simulink model "completed_microinverter_setup"  (R2022a)
settings: Solver=FixedStepDiscrete  StartTime=0.0  StopTime=2  FixedStep=Ts  RelTol=1e-3
InitFcn:
  | Ts=1e-6;
  | Tcs=1e-4;
values from neighbouring files (symbols this model uses):
  C1_filter = 2e-6    (= 2e-06)    [q4.m]
  C_filter = 100e-6    (= 0.0001)    [q1.m]    (also in q2.m; q4.m = 2e-06)
  f_center = 50    [q4.m]
  F_switch = 1e3    (= 1000)    [q1.m]
  Ki_current = L_filter*Wn^2    (= 15791.3670417)    [q1.m]    (also in q2.m = 63165.468167; q4.m = 493.480220054)
  Ki_pll = (Wn^2) / A    (= 394784.176044)    [q1.m]    (also in q4.m = 1579136.70417)
  Ki_power = 100    [q4.m]
  Ki_voltage = C_filter*Wn^2    (= 3.55305758439)    [q1.m]    (also in q4.m = 0.0710611516878)
  Kp_current = 2*L_filter*DF*Wn    (= 110.584061406)    [q1.m]    (also in q2.m = 71.0753921948; q4.m = 5.49778714378)
  Kp_pll = 2*DF / sqrt(A/Ki_pll)    [q1.m]    (also in q4.m = 2*DF / sqrt(1/Ki_pll))
  Kp_power = 0    [q4.m]
  Kp_voltage = 2*C_filter*DF*Wn    (= 0.0565486677646)    [q1.m]    (also in q4.m = 0.00791681348705)
  L1_filter = 1.5e-3    (= 0.0015)    [q4.m]
  L2_filter = 1.0e-3    (= 0.001)    [q4.m]
  L_filter = 40e-3    (= 0.04)    [q1.m]    (also in q2.m; q4.m = 0.00125)
  L_load = sqrt((R_load * V_rms^2)/P_load - R_load^2) / w    [q1.m]    (also in q4.m)
  R_load = (V_rms^2) * (pf_load^2) / P_load    (= 43.32)    [q1.m]    (also in q4.m)
  Rd_filter = 0.2    [q4.m]
  Tes = 20*Ts    (= 2e-05)    [q1.m]    (also in q4.m)
  V_dc = sqrt(2) * sqrt(3) * V_rms    [q1.m]    (also in q4.m = V_rms * sqrt(3) * sqrt(2))
undefined symbols (not defined in the file or in its folder): DiscIntNeverNeededParam
libraries: ee_lib x111, nesl_utility x28, fl_lib x23, spsabctodq0Lib x11, dspindex x3, spsTriangleGeneratorLib x2, spsdq0toabcLib x2
(part 1 of 4)
settings Model: VariantFading=off  Creator=Kevin  LastModifiedBy=acidi
settings SolverCC: AlgebraicLoopSolver=TrustRegion
settings DebuggingCC: UnconnectedInputMsg=warning  UnconnectedOutputMsg=warning  UnconnectedLineMsg=warning  SFMachineParentedDataDiag=warning

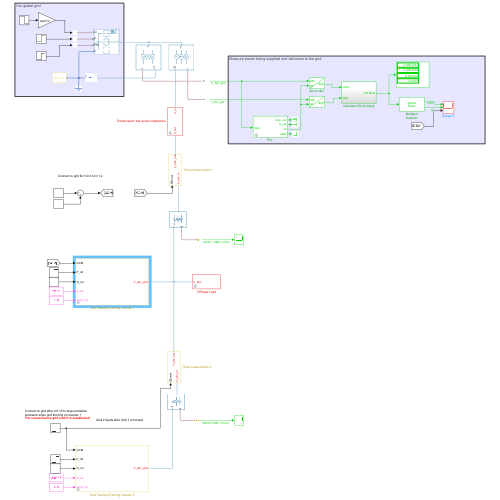
[thumbnail: Simulink's stored preview of the top-level diagram]
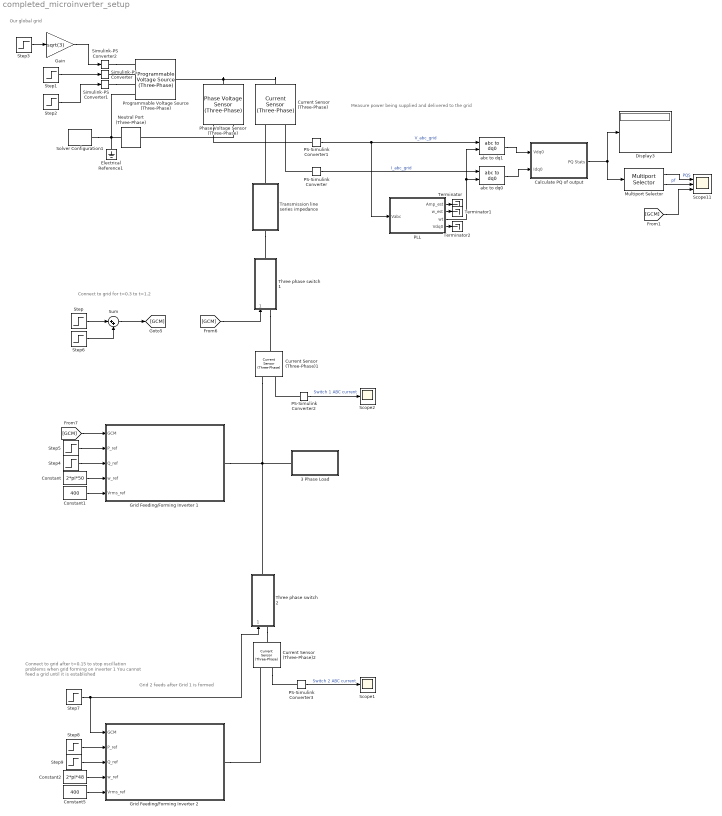
== system completed_microinverter_setup ==
  note: Grid 2 feeds after Grid 1 is formed
  note: Our global grid
  note: Measure power being supplied and delivered to the grid
  note: Connect to grid for t=0.3 to t=1.2
  note: Connect to grid after t=0.15 to stop oscillation problems when grid forming on inverter 1
      | You cannot feed a grid until it is established
  3 Phase Load : Subsystem  mask{R=R_load, L=L_load}
  Calculate PQ of output : Subsystem
  Constant : Constant  Value=2*pi*50
  Constant1 : Constant  Value=400
  Constant2 : Constant  Value=2*pi*48
  Constant5 : Constant  Value=400
  Current Sensor (Three-Phase) : ee_lib/Sensors & Transducers/Current Sensor (Three-Phase)
  Current Sensor (Three-Phase)1 : ee_lib/Sensors & Transducers/Current Sensor (Three-Phase)
  Current Sensor (Three-Phase)2 : ee_lib/Sensors & Transducers/Current Sensor (Three-Phase)
  Display3 : Display
  Electrical Reference1 : fl_lib/Electrical/Electrical Elements/Electrical Reference
      settings: SourceProductBaseCode=PW,SS,VE
  Gain : Gain  Gain=sqrt(3)
  Grid Feeding/Forming Inverter 1 : Subsystem  mask{Ts=Ts, Tes=Tes, Tcs=Tcs, Ki_pll=Ki_pll, Kp_pll=Kp_pll, f_center=f_center, L1_filter=L1_filter, L2_filter=L2_filter, C1_filter=C1_filter, Rd_filter=Rd_filter, C_filter=C_filter, L_filter=L_filter, Ki_current=Ki_current, Kp_current=Kp_current, Ki_voltage=Ki_voltage, Kp_voltage=Kp_voltage, Ki_power=Ki_power, Kp_power=Kp_power}
      mask DialogControl Container5 Prompt: Simulation constants
      mask DialogControl Container6 Prompt: Three Phase PLL
      mask DialogControl ParameterGroupVar Prompt: LCL inverter filter
      mask DialogControl Container3 Prompt: Controller Parameters
      mask DialogControl Container4 Prompt: Current controller
      mask DialogControl Container7 Prompt: Voltage Controller
      mask DialogControl Container8 Prompt: Power Controller
  Grid Feeding/Forming Inverter 2 : Subsystem  mask{Ts=Ts, Tes=Tes, Tcs=Tcs, Ki_pll=Ki_pll, Kp_pll=Kp_pll, f_center=f_center, L1_filter=L1_filter, L2_filter=L2_filter, C1_filter=C1_filter, Rd_filter=Rd_filter, C_filter=C_filter, L_filter=L_filter, Ki_current=Ki_current, Kp_current=Kp_current, Ki_voltage=Ki_voltage, Kp_voltage=Kp_voltage, Ki_power=Ki_power, Kp_power=Kp_power}
      mask DialogControl Container5 Prompt: Simulation constants
      mask DialogControl Container6 Prompt: Three Phase PLL
      mask DialogControl ParameterGroupVar Prompt: LCL inverter filter
      mask DialogControl Container3 Prompt: Controller Parameters
      mask DialogControl Container4 Prompt: Current controller
      mask DialogControl Container7 Prompt: Voltage Controller
      mask DialogControl Container8 Prompt: Power Controller
  Multiport Selector : dspindex/Multiport Selector  rowsOrCols=Rows  idxCellArray={ [1 2 3], 4 }  idxErrMode=Clip Index
  Neutral Port (Three-Phase) : ee_lib/Connectors & References/Neutral Port (Three-Phase)  G_parasitic=1e-12 1/Ohm
      settings: SourceProductBaseCode=PS  InternalSimscapePortConfiguration="{\"Bottom\":[],\"Left\":[{\"id\":\"N\",\"label\":\"~\",\"type\":\"foundation.electrical.three_phase\"}],\"Right\":[{\"id\":\"n\",\"label\":\"n\",\"type\":\"foundation.electrical.electrical\"}],\"Top\":[]}"
  PLL : Subsystem  mask{Ts=Tcs, Ki=Ki_pll, Kp=Kp_pll, f_center=f_center}
      mask DialogControl Container1 Prompt: Parameters
  PS-Simulink Converter{,1..3} (4 alike) : nesl_utility/PS-Simulink Converter  PhysicalDomain=network_engine_domain  SubClassName=ps_output  LeftPortType=input  RightPortType=output  PseudoPeriodic=off  Frequencies=[]  VectorFormat=inherit  Unit=inherit  AffineConversion=off
      settings: SourceProductBaseCode=SS,PW,VE
  Phase Voltage Sensor (Three-Phase) : ee_lib/Sensors & Transducers/Phase Voltage Sensor (Three-Phase)
      settings: SourceProductBaseCode=PS
  Programmable Voltage Source (Three-Phase) : ee_lib/Sources/Programmable Voltage Source (Three-Phase)  magnitude_type=ee.enum.timechanging.external  vline_rms=230*sqrt(3) V  magn_ramp=1 V/s  magn_step=-230*sqrt(3)*0.8 V  magn_modu_magn=1 V  magn_modu_freq=1 Hz  magn_t1=1.2 s  magn_t2=1.6 s  frequency_type=ee.enum.timechanging.external  freq=50 Hz  freq_ramp=1 Hz/s  freq_step=1 Hz  freq_modu_magn=1 Hz  freq_modu_freq=1 Hz  freq_t1=1 s  freq_t2=2 s  phase_type=ee.enum.timechanging.external  shift=45 deg  phase_ramp=1 deg/s  phase_step=15 deg  phase_modu_magn=1 deg  phase_modu_freq=1 Hz  phase_t1=0.5 s  phase_t2=0.9 s  impedance_option=1  SShortCircuit=1e6 V*A  XR=15  R=0.01 Ohm  L=3.97e-4 H  G_parasitic=0 1/Ohm  harmonic_option=0  harmonic_orders=[5, 7, 11, 13]  harmonic_ratios=[.1, .1, .1, .1]  harmonic_shifts=[0, 0, 0, 0] deg  harmonic_sequences=[1, 1, 1, 1]  harmonic_t1=-inf s  harmonic_t2=inf s  I_specify=off  I_priority=None  I=[ 0 0 0 ] A  I_nominal_specify=off  I_nominal_unit=A  I_nominal_value=1  V_specify=off  V_priority=None  V=[0, 400*sqrt(2/3)*sin(-2/3*pi), 400*sqrt(2/3)*sin(-4/3*pi)] V  V_nominal_specify=off  V_nominal_unit=V  V_nominal_value=1
      settings: SourceProductBaseCode=PS  InternalSimscapePortConfiguration="{\"Bottom\":[],\"Left\":[{\"id\":\"ext_magn\",\"label\":\"M\",\"type\":\"input\"},{\"id\":\"ext_freq\",\"label\":\"F\",\"type\":\"input\"},{\"id\":\"ext_phase\",\"label\":\"Phi\",\"type\":\"input\"},{\"id\":\"n\",\"label\":\"n\",\"type\":\"foundation.electrical.electrical\"}],\"Right\":[{\"id\":\"N\",\"label\":\"~\",\"type\":\"foundation.electrical.three_phase\"}],\"Top\":[]}"
  Scope1 : Scope
  Scope11 : Scope  NumInputPorts=3
  Scope2 : Scope
  Simulink-PS Converter : nesl_utility/Simulink-PS Converter  PhysicalDomain=network_engine_domain  SubClassName=ps_input  LeftPortType=input  RightPortType=output  PseudoPeriodic=off  Frequencies=[]  NoiseDistribution=none  NoiseParameters=[]  Unit=1  AffineConversion=off  FilteringAndDerivatives=provide  SimscapeFilterOrder=1  InputFilterTimeConstant=0.001  UdotUserProvided=0
      settings: SourceProductBaseCode=SS,PW,VE
  Simulink-PS Converter1 : nesl_utility/Simulink-PS Converter  PhysicalDomain=network_engine_domain  SubClassName=ps_input  LeftPortType=input  RightPortType=output  PseudoPeriodic=off  Frequencies=[]  NoiseDistribution=none  NoiseParameters=[]  Unit=1  AffineConversion=off  FilteringAndDerivatives=provide  SimscapeFilterOrder=1  InputFilterTimeConstant=0.001  UdotUserProvided=0
      settings: SourceProductBaseCode=SS,PW,VE
  Simulink-PS Converter2 : nesl_utility/Simulink-PS Converter  PhysicalDomain=network_engine_domain  SubClassName=ps_input  LeftPortType=input  RightPortType=output  PseudoPeriodic=off  Frequencies=[]  NoiseDistribution=none  NoiseParameters=[]  Unit=1  AffineConversion=off  FilteringAndDerivatives=provide  SimscapeFilterOrder=1  InputFilterTimeConstant=0.001  UdotUserProvided=0
      settings: SourceProductBaseCode=SS,PW,VE
  Solver Configuration1 : nesl_utility/Solver Configuration  PhysicalDomain=network_engine_domain  SubClassName=solver  LeftPortType=input  RightPortType=generic  Tones=[]  Harmonics=[]  SimulateNoise=off  Profile=off  UseLocalSampling=off  EnableSwitchedLinearOptims=on  FrequencyDomain=off  UseCCode=off  RelTol=0.001  AbsTol=1e-06  MinStep=1e-09  ToWorkspace=off  RevertToSquareIcSolve=off  NumHomotopyIterations=100  PhasorMode=off  PhasorModeNumHarmonics=1  IndexReductionMethod=DerivativeReplacement  DoDC=off  ResidualTolerance=1e-09  UseLocalSolver=on  LocalSolverChoice=NE_BACKWARD_EULER_ADVANCER  LocalSolverSampleTime=Tcs  DoFixedCost=off  MaxNonlinIter=3  MaxModeIter=2  ComputeImpulses=off  ImpulseIterations=2  LinearAlgebra=auto  LinearAlgebraNumThread=0  EquationFormulation=NE_TIME_EF  DelaysMemoryBudget=1024  AutomaticFiltering=off  FilteringTimeConstant=0.001  PartitionStorageMethod=AS_NEEDED  PartitionMemoryBudget=1024  PartitionMethod=ROBUST
      settings: SourceProductBaseCode=SS,PW,VE
  Step : Step  Time=0.3  SampleTime=0
  Step1 : Step  Time=0.4  Before=50  After=53  SampleTime=0
  Step2 : Step  Time=0.6  After=15 * pi/180  SampleTime=0
  Step3 : Step  Time=0.8  Before=400  After=400*0.6  SampleTime=0
  Step4 : Step  Time=0.5  Before=6000  After=-2000  SampleTime=0
  Step5 : Step  Time=0.7  Before=7000  After=15000  SampleTime=0
  Step6 : Step  Time=1.2  After=-1  SampleTime=0
  Step7 : Step  Time=0.15  SampleTime=0
  Step8 : Step  Time=1.4  Before=1000  After=15000  SampleTime=0
  Step9 : Step  Time=1.6  Before=-3000  After=4500  SampleTime=0
  Sum : Sum  Inputs=|++
  Terminator : Terminator
  Terminator1 : Terminator
  Terminator2 : Terminator
  Three phase switch 1 : Subsystem  mask{R_opened=1e9, R_closed=1e-3}
  Three phase switch 2 : Subsystem  mask{R_opened=1e9, R_closed=1e-3}
  Transmission line series impedance : Subsystem  mask{R=100e-3, L=1e-3}
  abc to dq0 : spsabctodq0Lib/abc to dq0  Alignment=90 degrees behind phase A axis
  abc to dq1 : spsabctodq0Lib/abc to dq0  Alignment=90 degrees behind phase A axis
  wires:
  Step1/1 -> Simulink-PS Converter/1
  Step2/1 -> Simulink-PS Converter1/1
  Step3/1 -> Gain/1
  Gain/1 -> Simulink-PS Converter2/1
  [GCM] -> Grid Feeding/Forming Inverter 1/1(GCM)
  Step5/1 -> Grid Feeding/Forming Inverter 1/2(P_ref)
  Step4/1 -> Grid Feeding/Forming Inverter 1/3(Q_ref)
  Constant/1 -> Grid Feeding/Forming Inverter 1/4(w_ref)
  Constant1/1 -> Grid Feeding/Forming Inverter 1/5(Vrms_ref)
  PS-Simulink Converter2/1 -> Scope2/1  "Switch 1 ABC current"
  [GCM] -> Three phase switch 1/1(Control)
  Step7/1 -> Grid Feeding/Forming Inverter 2/1(GCM), Three phase switch 2/1(Control)
  Step8/1 -> Grid Feeding/Forming Inverter 2/2(P_ref)
  Step9/1 -> Grid Feeding/Forming Inverter 2/3(Q_ref)
  Step/1 -> Sum/1
  Step6/1 -> Sum/2
  Constant2/1 -> Grid Feeding/Forming Inverter 2/4(w_ref)
  Constant5/1 -> Grid Feeding/Forming Inverter 2/5(Vrms_ref)
  Calculate PQ of output/1(PQ Stats) -> Multiport Selector/1, Display3/1
  Multiport Selector/1 -> Scope11/1  "PQS"
  Multiport Selector/2 -> Scope11/2  "pf"
  PS-Simulink Converter/1 -> abc to dq0/1  "I_abc_grid"
  PS-Simulink Converter1/1 -> PLL/1(Vabc), abc to dq1/1  "V_abc_grid"
  PLL/3(wt) -> abc to dq1/2, abc to dq0/2
  abc to dq1/1 -> Calculate PQ of output/1(Vdq0)
  abc to dq0/1 -> Calculate PQ of output/2(Idq0)
  [GCM] -> Scope11/3
  PLL/1(Amp_est) -> Terminator/1
  PLL/2(w_est) -> Terminator1/1
  PLL/4(Vdq0) -> Terminator2/1
  PS-Simulink Converter3/1 -> Scope1/1  "Switch 2 ABC current"
  Sum/1 -> [GCM]
  connections:
  Simulink-PS Converter/RConn1 -- Programmable Voltage Source (Three-Phase)/LConn2
  Simulink-PS Converter2/RConn1 -- Programmable Voltage Source (Three-Phase)/LConn1
  Programmable Voltage Source (Three-Phase)/LConn4 -- Electrical Reference1/LConn1 -- Neutral Port (Three-Phase)/RConn1 -- Solver Configuration1/RConn1
  Simulink-PS Converter1/RConn1 -- Programmable Voltage Source (Three-Phase)/LConn3
  Phase Voltage Sensor (Three-Phase)/LConn1 -- Current Sensor (Three-Phase)/LConn1 -- Programmable Voltage Source (Three-Phase)/RConn1
  Grid Feeding/Forming Inverter 1/RConn1 -- Three phase switch 2/RConn1 -- Current Sensor (Three-Phase)1/RConn2 -- 3 Phase Load/LConn1
  Transmission line series impedance/RConn1 -- Three phase switch 1/RConn1
  Grid Feeding/Forming Inverter 2/RConn1 -- Current Sensor (Three-Phase)2/RConn2
  Phase Voltage Sensor (Three-Phase)/RConn2 -- Neutral Port (Three-Phase)/LConn1
  Transmission line series impedance/LConn1 -- Current Sensor (Three-Phase)/RConn2
  PS-Simulink Converter/LConn1 -- Current Sensor (Three-Phase)/RConn1
  PS-Simulink Converter1/LConn1 -- Phase Voltage Sensor (Three-Phase)/RConn1
  Three phase switch 1/LConn1 -- Current Sensor (Three-Phase)1/LConn1
  PS-Simulink Converter2/LConn1 -- Current Sensor (Three-Phase)1/RConn1
  Three phase switch 2/LConn1 -- Current Sensor (Three-Phase)2/LConn1
  Current Sensor (Three-Phase)2/RConn1 -- PS-Simulink Converter3/LConn1

== system completed_microinverter_setup/3 Phase Load ==
  Inductor3 : ee_lib/Passive/Inductor  l=L H  enable_L_tol=0  L_tol=20  tol_distribution=1  nSigma=4  r=0 Ohm  g=1e-9 1/Ohm  enable_operating_limits=0  operating_limit_action=2  max_working_current=1 A  power_rating=1 W  enable_faults=0  fault_action=1  lambdaPercent=50  k_faulted=0.9999  turnsShort=0  openCct=0  groundShort=0  groundShortG=0 1/Ohm  tau_fault=1e-3 s  enable_temporal_fault=0  t_fault=1 s  enable_behavioral_fault=0  max_permissible_voltage=100 V  n_fail_on_voltage=1  max_permissible_current=1 A  t_fail_on_current=1 s  i_L_specify=off  i_L_priority=High  i_L=0 A  i_L_nominal_specify=off  i_L_nominal_unit=A  i_L_nominal_value=1
  Inductor4 : ee_lib/Passive/Inductor  l=L H  enable_L_tol=0  L_tol=20  tol_distribution=1  nSigma=4  r=0 Ohm  g=1e-9 1/Ohm  enable_operating_limits=0  operating_limit_action=2  max_working_current=1 A  power_rating=1 W  enable_faults=0  fault_action=1  lambdaPercent=50  k_faulted=0.9999  turnsShort=0  openCct=0  groundShort=0  groundShortG=0 1/Ohm  tau_fault=1e-3 s  enable_temporal_fault=0  t_fault=1 s  enable_behavioral_fault=0  max_permissible_voltage=100 V  n_fail_on_voltage=1  max_permissible_current=1 A  t_fail_on_current=1 s  i_L_specify=off  i_L_priority=High  i_L=0 A  i_L_nominal_specify=off  i_L_nominal_unit=A  i_L_nominal_value=1
  Inductor5 : ee_lib/Passive/Inductor  l=L H  enable_L_tol=0  L_tol=20  tol_distribution=1  nSigma=4  r=0 Ohm  g=1e-9 1/Ohm  enable_operating_limits=0  operating_limit_action=2  max_working_current=1 A  power_rating=1 W  enable_faults=0  fault_action=1  lambdaPercent=50  k_faulted=0.9999  turnsShort=0  openCct=0  groundShort=0  groundShortG=0 1/Ohm  tau_fault=1e-3 s  enable_temporal_fault=0  t_fault=1 s  enable_behavioral_fault=0  max_permissible_voltage=100 V  n_fail_on_voltage=1  max_permissible_current=1 A  t_fail_on_current=1 s  i_L_specify=off  i_L_priority=High  i_L=0 A  i_L_nominal_specify=off  i_L_nominal_unit=A  i_L_nominal_value=1
  Phase Splitter1 : ee_lib/Connectors & References/Phase Splitter
      settings: SourceProductBaseCode=PS
  Resistor : ee_lib/Passive/Resistor  R=R Ohm  enable_R_tol=0  R_tol=5  tol_distribution=1  nSigma=4  enable_operating_limits=0  operating_limit_action=2  max_working_voltage=100 V  power_rating=1 W  enable_faults=0  fault_action=1  R_faulted=inf Ohm  enable_temporal_fault=0  t_fault=1 s  enable_behavioral_fault=0  max_permissible_current=1 A  t_fail_on_current=1 s  noise_mode=0  sample_time=1e-3 s  repeatability=1  auto_seed=2348838240  user_seed=0  Tdevice=25 degC  power_derating_T1=70 degC  power_derating_T2=155 degC  operating_temperature_range_vec=[-50, 150] degC  alpha=3.93e-3 1/K  Tmeas=25 degC  thermal_mass=100 J/K  temperature_specify=off  temperature_priority=High  temperature=298.15 K  temperature_nominal_specify=off  temperature_nominal_unit=K  temperature_nominal_value=1
  Resistor1 : ee_lib/Passive/Resistor  R=R Ohm  enable_R_tol=0  R_tol=5  tol_distribution=1  nSigma=4  enable_operating_limits=0  operating_limit_action=2  max_working_voltage=100 V  power_rating=1 W  enable_faults=0  fault_action=1  R_faulted=inf Ohm  enable_temporal_fault=0  t_fault=1 s  enable_behavioral_fault=0  max_permissible_current=1 A  t_fail_on_current=1 s  noise_mode=0  sample_time=1e-3 s  repeatability=1  auto_seed=4112460543  user_seed=0  Tdevice=25 degC  power_derating_T1=70 degC  power_derating_T2=155 degC  operating_temperature_range_vec=[-50, 150] degC  alpha=3.93e-3 1/K  Tmeas=25 degC  thermal_mass=100 J/K  temperature_specify=off  temperature_priority=High  temperature=298.15 K  temperature_nominal_specify=off  temperature_nominal_unit=K  temperature_nominal_value=1
  Resistor2 : ee_lib/Passive/Resistor  R=R Ohm  enable_R_tol=0  R_tol=5  tol_distribution=1  nSigma=4  enable_operating_limits=0  operating_limit_action=2  max_working_voltage=100 V  power_rating=1 W  enable_faults=0  fault_action=1  R_faulted=inf Ohm  enable_temporal_fault=0  t_fault=1 s  enable_behavioral_fault=0  max_permissible_current=1 A  t_fail_on_current=1 s  noise_mode=0  sample_time=1e-3 s  repeatability=1  auto_seed=4144164703  user_seed=0  Tdevice=25 degC  power_derating_T1=70 degC  power_derating_T2=155 degC  operating_temperature_range_vec=[-50, 150] degC  alpha=3.93e-3 1/K  Tmeas=25 degC  thermal_mass=100 J/K  temperature_specify=off  temperature_priority=High  temperature=298.15 K  temperature_nominal_specify=off  temperature_nominal_unit=K  temperature_nominal_value=1
  V_abc : PMIOPort  Side=Left
  connections:
  Resistor2/LConn1 -- Inductor5/RConn1
  Phase Splitter1/RConn1 -- Inductor3/LConn1
  Phase Splitter1/RConn3 -- Inductor5/LConn1
  Resistor/RConn1 -- Resistor2/RConn1 -- Resistor1/RConn1
  Resistor1/LConn1 -- Inductor4/RConn1
  Phase Splitter1/RConn2 -- Inductor4/LConn1
  Resistor/LConn1 -- Inductor3/RConn1
  V_abc/RConn1 -- Phase Splitter1/LConn1

== system completed_microinverter_setup/Calculate PQ of output ==
  note: Reorient Vdq0 so that Uq = 0, Ud = defined
  Vdq0 : Inport
  Idq0 : Inport  Port=2
  Atan2 : Trigonometry  Operator=atan2
  Cos : Trigonometry  Operator=cos
  Demux : Demux  Outputs=3
  Demux1 : Demux  Outputs=2
  Gain2 : Gain  Gain=3/2
  MatrixMultiply1 : Product  Multiplication=Matrix(*)
  MatrixMultiply2 : Product  Multiplication=Matrix(*)
  Mux : Mux
  Product : Product
  Product2 : Product
  Selector : Selector  InputPortWidth=3  IndexOptions=Index vector (dialog)  Indices=[1 2]  OutputSizes=1
  Selector1 : Selector  InputPortWidth=3  IndexOptions=Index vector (dialog)  Indices=[1]  OutputSizes=1
  Sign : Signum
  Sqrt : Sqrt
  Square : Math  Operator=square
  Subsystem : Subsystem
  Sum of Elements : Sum  Inputs=+
  Terminator : Terminator
  PQ Stats : Outport
  wires:
  Product2/1 -> Gain2/1
  Square/1 -> Sum of Elements/1
  Gain2/1 -> Demux/1, Selector/1
  Sum of Elements/1 -> Sqrt/1
  Selector/1 -> Square/1, Demux1/1
  Vdq0/1 -> MatrixMultiply1/2, Subsystem/1(Vdq0)
  Subsystem/1(Rotation Matrix) -> MatrixMultiply2/1, MatrixMultiply1/1
  Idq0/1 -> MatrixMultiply2/2
  MatrixMultiply1/1 -> Selector1/1
  MatrixMultiply2/1 -> Product2/2
  Demux/3 -> Terminator/1
  Demux/2 -> Atan2/1  "Q"
  Demux/1 -> Atan2/2  "P"
  Atan2/1 -> Cos/1
  Demux1/1 -> Mux/1  "P"
  Demux1/2 -> Sign/1, Mux/2  "Q"
  Sqrt/1 -> Mux/3  "|S|"
  Product/1 -> Mux/4  "pf"
  Mux/1 -> PQ Stats/1
  Selector1/1 -> Product2/1
  Sign/1 -> Product/1
  Cos/1 -> Product/2  "pf"

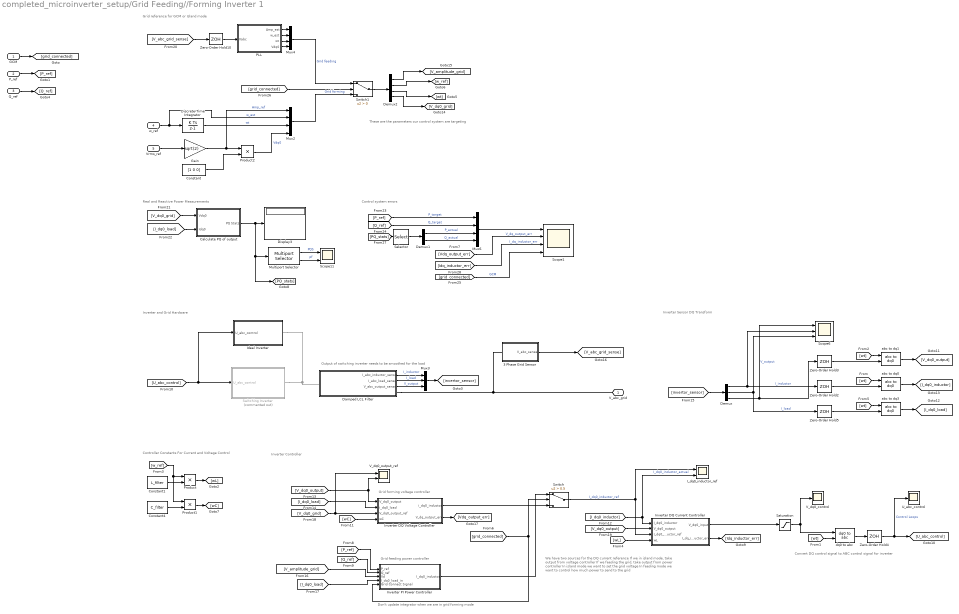
== system completed_microinverter_setup/Grid Feeding//Forming Inverter 1 ==
  note: Grid forming voltage controller
  note: Output of switching inverter needs to be smoothed for the load
  note: These are the parameters our control system are targeting
  note: Don't update integrator when we are in grid forming mode
  note: We have two sources for the DQ current reference
      | If we in island mode, take output from voltage controller
      | If we feeding the grid, take output from power controller
      |
      | In island mode we want to set the grid voltage
      | In feeding mode we want to control how much power to send to the grid
  note: Convert DQ control signal to ABC control signal for inverter
  note: Control system errors
  note: Grid reference for GCM or Island mode
  note: Real and Reactive Power Measurements
  note: Inverter and Grid Hardware
  note: Inverter Sensor DQ Transform
  note: Inverter Controller
  note: Controller Constants For Current and Voltage Control
  note: Grid feeding power controller
  GCM : Inport
  P_ref : Inport  Port=2
  Q_ref : Inport  Port=3
  w_ref : Inport  Port=4
  Vrms_ref : Inport  Port=5
  3 Phase Grid Sensor : Subsystem  mask{R=10e3}
  Calculate PQ of output : Subsystem
  Constant : Constant  Value=[1 0 0]
  Constant1 : Constant  Value=L_filter
  Constant4 : Constant  Value=C_filter
  Damped LCL Filter : Subsystem  mask{L1=L1_filter, L2=L2_filter, C=C1_filter, Rd=Rd_filter, Ts=Tcs}
  Demux : Demux  Outputs=3
  Demux1 : Demux  Outputs=2
  Demux2 : Demux
  Discrete-Time Integrator : DiscreteIntegrator  SampleTime=Tcs  UpperSaturationLimit=2*pi*10  LowerSaturationLimit=-2*pi*10  ICPrevOutput=DiscIntNeverNeededParam  ICPrevScaledInput=DiscIntNeverNeededParam
  Display3 : Display
  Gain : Gain  Gain=sqrt(2)
  I_dq0_inductor_ref : Scope  NumInputPorts=2
  Ideal Inverter : Subsystem
  Inverter DQ Current Controller : Subsystem  mask{Kp=Kp_current, Ki=Ki_current, Ts=Tcs}
  Inverter DQ Voltage Controller : Subsystem  mask{Kp=Kp_voltage, Ki=Ki_voltage, Ts=Tcs}
  Inverter PI Power Controller : Subsystem  mask{Ki=Ki_power, Kp=Kp_power, Ts=Tcs}
  Multiport Selector : dspindex/Multiport Selector  rowsOrCols=Rows  idxCellArray={ [1 2 3], 4 }  idxErrMode=Clip Index
  Mux2 : Mux
  Mux3 : Mux  Inputs=3
  Mux4 : Mux
  Mux6 : Mux
  PLL : Subsystem  mask{Ts=Tcs, Ki=Ki_pll, Kp=Kp_pll, f_center=f_center}
      mask DialogControl Container1 Prompt: Parameters
  Product : Product
  Product1 : Product
  Product2 : Product
  Saturation : Saturate  UpperLimit=600  LowerLimit=-600
  Scope1 : Scope  NumInputPorts=4
  Scope11 : Scope  NumInputPorts=2
  Scope6 : Scope  NumInputPorts=3
  Selector : Selector  InputPortWidth=4  IndexOptions=Index vector (dialog)  Indices=[1 2]  OutputSizes=1
  Switch : Switch  Criteria=u2 > Threshold  Threshold=0.5  SaturateOnIntegerOverflow=off  InputSameDT=off
  Switch1 : Switch  Criteria=u2 > Threshold  SaturateOnIntegerOverflow=off  InputSameDT=off
  Switching Inverter : Subsystem  Commented=on  TreatAsAtomicUnit=on  mask{V_dc=V_dc, F_switch=F_switch, Ts=Tes}
  U_abc_control : Scope
  V_dq0_control : Scope
  V_dq0_output_ref : Scope  NumInputPorts=2
  Zero-Order Hold{2..5,10} (5 alike) : ZeroOrderHold  SampleTime=Tcs
  abc to dq0 : spsabctodq0Lib/abc to dq0  Alignment=Aligned with phase A axis
  abc to dq1 : spsabctodq0Lib/abc to dq0  Alignment=Aligned with phase A axis
  abc to dq3 : spsabctodq0Lib/abc to dq0  Alignment=Aligned with phase A axis
  dq0 to abc : spsdq0toabcLib/dq0 to abc  Alignment=Aligned with phase A axis
  V_abc_grid : PMIOPort  Side=Right
  wires:
  abc to dq1/1 -> [V_dq0_output]
  [w_ref] -> Product/1, Product1/1
  Constant1/1 -> Product/2
  Product1/1 -> [wC]
  [wt] -> abc to dq1/2
  Zero-Order Hold4/1 -> [U_abc_control], U_abc_control/1  "Control Loops"
  [wC] -> Inverter DQ Voltage Controller/4(wC)
  Switch/1 -> I_dq0_inductor_ref/1, Inverter DQ Current Controller/3(I_dq0_inductor_ref)  "I_dq0_inductor_ref"
  Inverter DQ Current Controller/1(V_dq0_input) -> Saturation/1
  [wt] -> dq0 to abc/2
  Constant4/1 -> Product1/2
  [wL] -> Inverter DQ Current Controller/4(wL)
  Product/1 -> [wL]
  dq0 to abc/1 -> Zero-Order Hold4/1
  [wt] -> abc to dq0/2
  [wt] -> abc to dq3/2
  Demux/2 -> Scope6/3, Zero-Order Hold5/1  "I_load"
  Demux/1 -> Scope6/2, Zero-Order Hold2/1  "I_inductor"
  Demux/3 -> Scope6/1, Zero-Order Hold3/1  "V_output"
  Zero-Order Hold10/1 -> PLL/1(Vabc)
  Saturation/1 -> dq0 to abc/1, V_dq0_control/1
  Zero-Order Hold2/1 -> abc to dq0/1
  Damped LCL Filter/1(I_abc_inductor_sense) -> Mux3/1  "I_inductor"
  Damped LCL Filter/2(I_abc_load_sense) -> Mux3/2  "I_load"
  Damped LCL Filter/3(V_abc_output_sense) -> Mux3/3  "V_output"
  Mux3/1 -> [invertor_sensor]
  Zero-Order Hold5/1 -> abc to dq3/1
  [grid_connected] -> Switch/2, Inverter PI Power Controller/5(Grid Connect Signal)
  [P_ref] -> Inverter PI Power Controller/1(P_ref)
  [Q_ref] -> Inverter PI Power Controller/2(Q_ref)
  Calculate PQ of output/1(PQ Stats) -> [PQ_stats], Multiport Selector/1, Display3/1
  Zero-Order Hold3/1 -> abc to dq1/1
  [U_abc_control] -> Ideal Inverter/1(U_abc_control), Switching Inverter/1(U_abc_control)
  [V_dq0_output] -> Inverter DQ Voltage Controller/1(V_dq0_output), V_dq0_output_ref/2
  abc to dq3/1 -> [I_dq0_load]
  abc to dq0/1 -> [I_dq0_inductor]
  [V_amplitude_grid] -> Inverter PI Power Controller/3(Vd)
  [I_dq0_load] -> Inverter PI Power Controller/4(I_dq0_load_in)
  [V_dq0_grid] -> V_dq0_output_ref/1, Inverter DQ Voltage Controller/3(V_dq0_output_ref)
  [I_dq0_load] -> Inverter DQ Voltage Controller/2(i_dq0_load)
  [I_dq0_inductor] -> I_dq0_inductor_ref/2, Inverter DQ Current Controller/1(I_dq0_inductor)  "I_dq0_inductor_actual"
  [V_dq0_output] -> Inverter DQ Current Controller/2(V_dq0_output)
  3 Phase Grid Sensor/1(V_abc_sense) -> [V_abc_grid_sense]
  [V_abc_grid_sense] -> Zero-Order Hold10/1
  [V_dq0_grid] -> Calculate PQ of output/1(Vdq0)
  [I_dq0_load] -> Calculate PQ of output/2(Idq0)
  [invertor_sensor] -> Demux/1
  GCM/1 -> [grid_connected]
  Q_ref/1 -> [Q_ref]
  P_ref/1 -> [P_ref]
  Multiport Selector/1 -> Scope11/1  "PQS"
  Multiport Selector/2 -> Scope11/2  "pf"
  w_ref/1 -> Discrete-Time Integrator/1, Mux2/2  "w_est"
  Discrete-Time Integrator/1 -> Mux2/3  "wt"
  Demux2/1 -> [V_amplitude_grid]
  Demux2/4 -> [V_dq0_grid]
  Demux2/3 -> [wt]
  Demux2/2 -> [w_ref]
  Vrms_ref/1 -> Gain/1
  Gain/1 -> Product2/1, Mux2/1  "Amp_ref"
  Constant/1 -> Product2/2
  Product2/1 -> Mux2/4  "Vdq0"
  PLL/1(Amp_est) -> Mux4/1
  PLL/2(w_est) -> Mux4/2
  PLL/3(wt) -> Mux4/3
  PLL/4(Vdq0) -> Mux4/4
  Switch1/1 -> Demux2/1
  Mux4/1 -> Switch1/1  "Grid feeding"
  [grid_connected] -> Switch1/2
  Mux2/1 -> Switch1/3  "Grid forming"
  [grid_connected] -> Scope1/4  "GCM"
  [PQ_stats] -> Selector/1
  Selector/1 -> Demux1/1
  [P_ref] -> Mux6/1  "P_target"
  [Q_ref] -> Mux6/2  "Q_target"
  Demux1/1 -> Mux6/3  "P_actual"
  Demux1/2 -> Mux6/4  "Q_actual"
  Mux6/1 -> Scope1/1
  [Vdq_output_err] -> Scope1/2  "V_dq_output_err"
  [Idq_inductor_err] -> Scope1/3  "I_dq_inductor_err"
  Inverter DQ Current Controller/2(I_dq_inductor_err) -> [Idq_inductor_err]
  Inverter DQ Voltage Controller/2(V_dq_output_err) -> [Vdq_output_err]
  Inverter PI Power Controller/1(I_dq0_inductor) -> Switch/1
  Inverter DQ Voltage Controller/1(i_dq0_inductor) -> Switch/3
  connections:
  Switching Inverter/RConn1 -- Ideal Inverter/RConn1 -- Damped LCL Filter/LConn1
  3 Phase Grid Sensor/LConn1 -- V_abc_grid/RConn1 -- Damped LCL Filter/RConn1

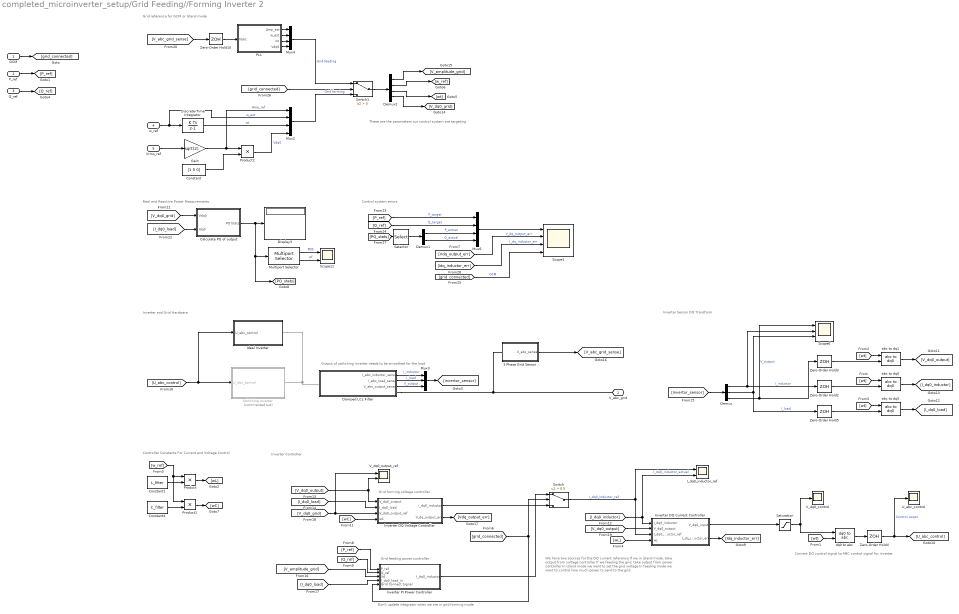
== system completed_microinverter_setup/Grid Feeding//Forming Inverter 2 ==
  note: Grid forming voltage controller
  note: Output of switching inverter needs to be smoothed for the load
  note: These are the parameters our control system are targeting
  note: Don't update integrator when we are in grid forming mode
  note: We have two sources for the DQ current reference
      | If we in island mode, take output from voltage controller
      | If we feeding the grid, take output from power controller
      |
      | In island mode we want to set the grid voltage
      | In feeding mode we want to control how much power to send to the grid
  note: Convert DQ control signal to ABC control signal for inverter
  note: Control system errors
  note: Grid reference for GCM or Island mode
  note: Real and Reactive Power Measurements
  note: Inverter and Grid Hardware
  note: Inverter Sensor DQ Transform
  note: Inverter Controller
  note: Controller Constants For Current and Voltage Control
  note: Grid feeding power controller
  GCM : Inport
  P_ref : Inport  Port=2
  Q_ref : Inport  Port=3
  w_ref : Inport  Port=4
  Vrms_ref : Inport  Port=5
  3 Phase Grid Sensor : Subsystem  mask{R=10e3}
  Calculate PQ of output : Subsystem
  Constant : Constant  Value=[1 0 0]
  Constant1 : Constant  Value=L_filter
  Constant4 : Constant  Value=C_filter
  Damped LCL Filter : Subsystem  mask{L1=L1_filter, L2=L2_filter, C=C1_filter, Rd=Rd_filter, Ts=Tcs}
  Demux : Demux  Outputs=3
  Demux1 : Demux  Outputs=2
  Demux2 : Demux
  Discrete-Time Integrator : DiscreteIntegrator  SampleTime=Tcs  UpperSaturationLimit=2*pi*10  LowerSaturationLimit=-2*pi*10  ICPrevOutput=DiscIntNeverNeededParam  ICPrevScaledInput=DiscIntNeverNeededParam
  Display3 : Display
  Gain : Gain  Gain=sqrt(2)
  I_dq0_inductor_ref : Scope  NumInputPorts=2
  Ideal Inverter : Subsystem
  Inverter DQ Current Controller : Subsystem  mask{Kp=Kp_current, Ki=Ki_current, Ts=Tcs}
  Inverter DQ Voltage Controller : Subsystem  mask{Kp=Kp_voltage, Ki=Ki_voltage, Ts=Tcs}
  Inverter PI Power Controller : Subsystem  mask{Ki=Ki_power, Kp=Kp_power, Ts=Tcs}
  Multiport Selector : dspindex/Multiport Selector  rowsOrCols=Rows  idxCellArray={ [1 2 3], 4 }  idxErrMode=Clip Index
  Mux2 : Mux
  Mux3 : Mux  Inputs=3
  Mux4 : Mux
  Mux6 : Mux
  PLL : Subsystem  mask{Ts=Tcs, Ki=Ki_pll, Kp=Kp_pll, f_center=f_center}
      mask DialogControl Container1 Prompt: Parameters
  Product : Product
  Product1 : Product
  Product2 : Product
  Saturation : Saturate  UpperLimit=600  LowerLimit=-600
  Scope1 : Scope  NumInputPorts=4
  Scope11 : Scope  NumInputPorts=2
  Scope6 : Scope  NumInputPorts=3
  Selector : Selector  InputPortWidth=4  IndexOptions=Index vector (dialog)  Indices=[1 2]  OutputSizes=1
  Switch : Switch  Criteria=u2 > Threshold  Threshold=0.5  SaturateOnIntegerOverflow=off  InputSameDT=off
  Switch1 : Switch  Criteria=u2 > Threshold  SaturateOnIntegerOverflow=off  InputSameDT=off
  Switching Inverter : Subsystem  Commented=on  TreatAsAtomicUnit=on  mask{V_dc=V_dc, F_switch=F_switch, Ts=Tes}
  U_abc_control : Scope
  V_dq0_control : Scope
  V_dq0_output_ref : Scope  NumInputPorts=2
  Zero-Order Hold{2..5,10} (5 alike) : ZeroOrderHold  SampleTime=Tcs
  abc to dq0 : spsabctodq0Lib/abc to dq0  Alignment=Aligned with phase A axis
  abc to dq1 : spsabctodq0Lib/abc to dq0  Alignment=Aligned with phase A axis
  abc to dq3 : spsabctodq0Lib/abc to dq0  Alignment=Aligned with phase A axis
  dq0 to abc : spsdq0toabcLib/dq0 to abc  Alignment=Aligned with phase A axis
  V_abc_grid : PMIOPort  Side=Right
  wires:
  abc to dq1/1 -> [V_dq0_output]
  [w_ref] -> Product/1, Product1/1
  Constant1/1 -> Product/2
  Product1/1 -> [wC]
  [wt] -> abc to dq1/2
  Zero-Order Hold4/1 -> [U_abc_control], U_abc_control/1  "Control Loops"
  [wC] -> Inverter DQ Voltage Controller/4(wC)
  Switch/1 -> I_dq0_inductor_ref/1, Inverter DQ Current Controller/3(I_dq0_inductor_ref)  "I_dq0_inductor_ref"
  Inverter DQ Current Controller/1(V_dq0_input) -> Saturation/1
  [wt] -> dq0 to abc/2
  Constant4/1 -> Product1/2
  [wL] -> Inverter DQ Current Controller/4(wL)
  Product/1 -> [wL]
  dq0 to abc/1 -> Zero-Order Hold4/1
  [wt] -> abc to dq0/2
  [wt] -> abc to dq3/2
  Demux/2 -> Scope6/3, Zero-Order Hold5/1  "I_load"
  Demux/1 -> Scope6/2, Zero-Order Hold2/1  "I_inductor"
  Demux/3 -> Scope6/1, Zero-Order Hold3/1  "V_output"
  Zero-Order Hold10/1 -> PLL/1(Vabc)
  Saturation/1 -> dq0 to abc/1, V_dq0_control/1
  Zero-Order Hold2/1 -> abc to dq0/1
  Damped LCL Filter/1(I_abc_inductor_sense) -> Mux3/1  "I_inductor"
  Damped LCL Filter/2(I_abc_load_sense) -> Mux3/2  "I_load"
  Damped LCL Filter/3(V_abc_output_sense) -> Mux3/3  "V_output"
  Mux3/1 -> [invertor_sensor]
  Zero-Order Hold5/1 -> abc to dq3/1
  [grid_connected] -> Switch/2, Inverter PI Power Controller/5(Grid Connect Signal)
  [P_ref] -> Inverter PI Power Controller/1(P_ref)
  [Q_ref] -> Inverter PI Power Controller/2(Q_ref)
  Calculate PQ of output/1(PQ Stats) -> [PQ_stats], Multiport Selector/1, Display3/1
  Zero-Order Hold3/1 -> abc to dq1/1
  [U_abc_control] -> Ideal Inverter/1(U_abc_control), Switching Inverter/1(U_abc_control)
  [V_dq0_output] -> Inverter DQ Voltage Controller/1(V_dq0_output), V_dq0_output_ref/2
  abc to dq3/1 -> [I_dq0_load]
  abc to dq0/1 -> [I_dq0_inductor]
  [V_amplitude_grid] -> Inverter PI Power Controller/3(Vd)
  [I_dq0_load] -> Inverter PI Power Controller/4(I_dq0_load_in)
  [V_dq0_grid] -> V_dq0_output_ref/1, Inverter DQ Voltage Controller/3(V_dq0_output_ref)
  [I_dq0_load] -> Inverter DQ Voltage Controller/2(i_dq0_load)
  [I_dq0_inductor] -> I_dq0_inductor_ref/2, Inverter DQ Current Controller/1(I_dq0_inductor)  "I_dq0_inductor_actual"
  [V_dq0_output] -> Inverter DQ Current Controller/2(V_dq0_output)
  3 Phase Grid Sensor/1(V_abc_sense) -> [V_abc_grid_sense]
  [V_abc_grid_sense] -> Zero-Order Hold10/1
  [V_dq0_grid] -> Calculate PQ of output/1(Vdq0)
  [I_dq0_load] -> Calculate PQ of output/2(Idq0)
  [invertor_sensor] -> Demux/1
  GCM/1 -> [grid_connected]
  Q_ref/1 -> [Q_ref]
  P_ref/1 -> [P_ref]
  Multiport Selector/1 -> Scope11/1  "PQS"
  Multiport Selector/2 -> Scope11/2  "pf"
  w_ref/1 -> Discrete-Time Integrator/1, Mux2/2  "w_est"
  Discrete-Time Integrator/1 -> Mux2/3  "wt"
  Demux2/1 -> [V_amplitude_grid]
  Demux2/4 -> [V_dq0_grid]
  Demux2/3 -> [wt]
  Demux2/2 -> [w_ref]
  Vrms_ref/1 -> Gain/1
  Gain/1 -> Product2/1, Mux2/1  "Amp_ref"
  Constant/1 -> Product2/2
  Product2/1 -> Mux2/4  "Vdq0"
  PLL/1(Amp_est) -> Mux4/1
  PLL/2(w_est) -> Mux4/2
  PLL/3(wt) -> Mux4/3
  PLL/4(Vdq0) -> Mux4/4
  Switch1/1 -> Demux2/1
  Mux4/1 -> Switch1/1  "Grid feeding"
  [grid_connected] -> Switch1/2
  Mux2/1 -> Switch1/3  "Grid forming"
  [grid_connected] -> Scope1/4  "GCM"
  [PQ_stats] -> Selector/1
  Selector/1 -> Demux1/1
  [P_ref] -> Mux6/1  "P_target"
  [Q_ref] -> Mux6/2  "Q_target"
  Demux1/1 -> Mux6/3  "P_actual"
  Demux1/2 -> Mux6/4  "Q_actual"
  Mux6/1 -> Scope1/1
  [Vdq_output_err] -> Scope1/2  "V_dq_output_err"
  [Idq_inductor_err] -> Scope1/3  "I_dq_inductor_err"
  Inverter DQ Current Controller/2(I_dq_inductor_err) -> [Idq_inductor_err]
  Inverter DQ Voltage Controller/2(V_dq_output_err) -> [Vdq_output_err]
  Inverter PI Power Controller/1(I_dq0_inductor) -> Switch/1
  Inverter DQ Voltage Controller/1(i_dq0_inductor) -> Switch/3
  connections:
  Switching Inverter/RConn1 -- Ideal Inverter/RConn1 -- Damped LCL Filter/LConn1
  3 Phase Grid Sensor/LConn1 -- Damped LCL Filter/RConn1 -- V_abc_grid/RConn1

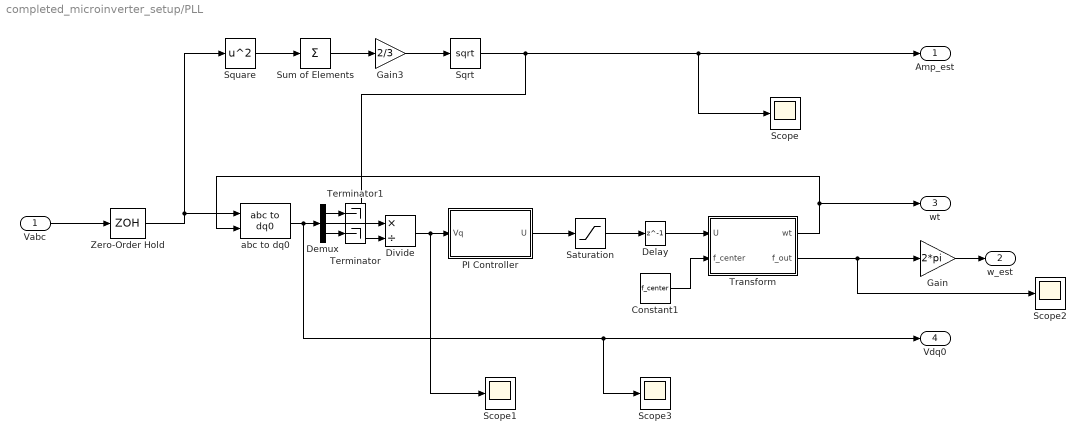
== system completed_microinverter_setup/PLL ==
  Vabc : Inport
  Constant1 : Constant  Value=f_center
  Delay : Delay  DelayLength=1  SampleTime=Ts
  Demux : Demux  Outputs=3
  Divide : Product  Inputs=*/
  Gain : Gain  Gain=2*pi
  Gain3 : Gain  Gain=2/3
  PI Controller : Subsystem
  Saturation : Saturate  UpperLimit=2*pi*4.8  LowerLimit=-2*pi*4.8
  Scope{,1..3} (4 alike) : Scope
  Sqrt : Sqrt
  Square : Math  Operator=square
  Sum of Elements : Sum  Inputs=+
  Terminator : Terminator
  Terminator1 : Terminator
  Transform : Subsystem
  Zero-Order Hold : ZeroOrderHold  SampleTime=Ts
  abc to dq0 : spsabctodq0Lib/abc to dq0  Alignment=Aligned with phase A axis
  Amp_est : Outport
  w_est : Outport  Port=2
  wt : Outport  Port=3
  Vdq0 : Outport  Port=4
  wires:
  Square/1 -> Sum of Elements/1
  Sum of Elements/1 -> Gain3/1
  Gain3/1 -> Sqrt/1
  Constant1/1 -> Transform/2(f_center)
  Divide/1 -> Scope1/1, PI Controller/1(Vq)
  PI Controller/1(U) -> Saturation/1
  Sqrt/1 -> Divide/2, Scope/1, Amp_est/1
  Transform/2(f_out) -> Scope2/1, Gain/1
  Transform/1(wt) -> abc to dq0/2, wt/1
  Zero-Order Hold/1 -> abc to dq0/1, Square/1
  Saturation/1 -> Delay/1
  Delay/1 -> Transform/1(U)
  Vabc/1 -> Zero-Order Hold/1
  abc to dq0/1 -> Scope3/1, Vdq0/1, Demux/1
  Demux/2 -> Divide/1
  Gain/1 -> w_est/1
  Demux/3 -> Terminator/1
  Demux/1 -> Terminator1/1

== system completed_microinverter_setup/Three phase switch 1 ==
  Control : Inport
  Controlled Voltage Source : fl_lib/Electrical/Electrical Sources/Controlled Voltage Source
      settings: SourceProductBaseCode=PW,SS,VE
  Electrical Reference : fl_lib/Electrical/Electrical Elements/Electrical Reference
      settings: SourceProductBaseCode=PW,SS,VE
  Phase Splitter : ee_lib/Connectors & References/Phase Splitter
      settings: SourceProductBaseCode=PS
  Phase Splitter1 : ee_lib/Connectors & References/Phase Splitter
      settings: SourceProductBaseCode=PS
  Simulink-PS Converter3 : nesl_utility/Simulink-PS Converter  PhysicalDomain=network_engine_domain  SubClassName=ps_input  LeftPortType=input  RightPortType=output  PseudoPeriodic=off  Frequencies=[]  NoiseDistribution=none  NoiseParameters=[]  Unit=1  AffineConversion=off  FilteringAndDerivatives=provide  SimscapeFilterOrder=1  InputFilterTimeConstant=0.001  UdotUserProvided=0
      settings: SourceProductBaseCode=SS,PW,VE
  Voltage-Controlled Switch : ee_lib/Additional Components/SPICE Passives/Voltage-Controlled Switch  SWITCH_model=ee.enum.switches.switchModelVoltage.resistance  VON=0.7 V  VOFF=0.3 V  VT=0 V  VH=0 V  RON=R_closed Ohm  ROFF_res=R_opened Ohm  Roff_gmin=ee.enum.switches.offResistance.no  ROFF=1e12 Ohm  TD=0 s
      settings: SourceProductBaseCode=PS  InternalSimscapePortConfiguration="{\"Bottom\":[],\"Left\":[{\"id\":\"p1\",\"label\":\"1+\",\"type\":\"foundation.electrical.electrical\"},{\"id\":\"p2\",\"label\":\"2+\",\"type\":\"foundation.electrical.electrical\"}],\"Right\":[{\"id\":\"n1\",\"label\":\"1-\",\"type\":\"foundation.electrical.electrical\"},{\"id\":\"n2\",\"label\":\"2-\",\"type\":\"foundation.electrical.electrical\"}],\"Top\":[]}"
  Voltage-Controlled Switch1 : ee_lib/Additional Components/SPICE Passives/Voltage-Controlled Switch  SWITCH_model=ee.enum.switches.switchModelVoltage.resistance  VON=0.7 V  VOFF=0.3 V  VT=0 V  VH=0 V  RON=R_closed Ohm  ROFF_res=R_opened Ohm  Roff_gmin=ee.enum.switches.offResistance.no  ROFF=1e12 Ohm  TD=0 s
      settings: SourceProductBaseCode=PS  InternalSimscapePortConfiguration="{\"Bottom\":[],\"Left\":[{\"id\":\"p1\",\"label\":\"1+\",\"type\":\"foundation.electrical.electrical\"},{\"id\":\"p2\",\"label\":\"2+\",\"type\":\"foundation.electrical.electrical\"}],\"Right\":[{\"id\":\"n1\",\"label\":\"1-\",\"type\":\"foundation.electrical.electrical\"},{\"id\":\"n2\",\"label\":\"2-\",\"type\":\"foundation.electrical.electrical\"}],\"Top\":[]}"
  Voltage-Controlled Switch2 : ee_lib/Additional Components/SPICE Passives/Voltage-Controlled Switch  SWITCH_model=ee.enum.switches.switchModelVoltage.resistance  VON=0.7 V  VOFF=0.3 V  VT=0 V  VH=0 V  RON=R_closed Ohm  ROFF_res=R_opened Ohm  Roff_gmin=ee.enum.switches.offResistance.no  ROFF=1e12 Ohm  TD=0 s
      settings: SourceProductBaseCode=PS  InternalSimscapePortConfiguration="{\"Bottom\":[],\"Left\":[{\"id\":\"p1\",\"label\":\"1+\",\"type\":\"foundation.electrical.electrical\"},{\"id\":\"p2\",\"label\":\"2+\",\"type\":\"foundation.electrical.electrical\"}],\"Right\":[{\"id\":\"n1\",\"label\":\"1-\",\"type\":\"foundation.electrical.electrical\"},{\"id\":\"n2\",\"label\":\"2-\",\"type\":\"foundation.electrical.electrical\"}],\"Top\":[]}"
  V_abc_in : PMIOPort  Side=Left
  V_abc_out : PMIOPort  Port=2  Side=Right
  wires:
  Control/1 -> Simulink-PS Converter3/1
  connections:
  Voltage-Controlled Switch/LConn1 -- Voltage-Controlled Switch2/LConn1 -- Voltage-Controlled Switch1/LConn1 -- Controlled Voltage Source/LConn1
  Voltage-Controlled Switch/RConn1 -- Controlled Voltage Source/RConn2 -- Electrical Reference/LConn1 -- Voltage-Controlled Switch1/RConn1 -- Voltage-Controlled Switch2/RConn1
  Simulink-PS Converter3/RConn1 -- Controlled Voltage Source/RConn1
  Voltage-Controlled Switch/RConn2 -- Phase Splitter/RConn1
  Phase Splitter1/RConn1 -- Voltage-Controlled Switch/LConn2
  V_abc_out/RConn1 -- Phase Splitter1/LConn1
  Voltage-Controlled Switch1/LConn2 -- Phase Splitter1/RConn2
  Voltage-Controlled Switch2/LConn2 -- Phase Splitter1/RConn3
  Voltage-Controlled Switch1/RConn2 -- Phase Splitter/RConn2
  Phase Splitter/LConn1 -- V_abc_in/RConn1
  Voltage-Controlled Switch2/RConn2 -- Phase Splitter/RConn3

== system completed_microinverter_setup/Three phase switch 2 ==
  Control : Inport
  Controlled Voltage Source : fl_lib/Electrical/Electrical Sources/Controlled Voltage Source
      settings: SourceProductBaseCode=PW,SS,VE
  Electrical Reference : fl_lib/Electrical/Electrical Elements/Electrical Reference
      settings: SourceProductBaseCode=PW,SS,VE
  Phase Splitter : ee_lib/Connectors & References/Phase Splitter
      settings: SourceProductBaseCode=PS
  Phase Splitter1 : ee_lib/Connectors & References/Phase Splitter
      settings: SourceProductBaseCode=PS
  Simulink-PS Converter3 : nesl_utility/Simulink-PS Converter  PhysicalDomain=network_engine_domain  SubClassName=ps_input  LeftPortType=input  RightPortType=output  PseudoPeriodic=off  Frequencies=[]  NoiseDistribution=none  NoiseParameters=[]  Unit=1  AffineConversion=off  FilteringAndDerivatives=provide  SimscapeFilterOrder=1  InputFilterTimeConstant=0.001  UdotUserProvided=0
      settings: SourceProductBaseCode=SS,PW,VE
  Voltage-Controlled Switch : ee_lib/Additional Components/SPICE Passives/Voltage-Controlled Switch  SWITCH_model=ee.enum.switches.switchModelVoltage.resistance  VON=0.7 V  VOFF=0.3 V  VT=0 V  VH=0 V  RON=R_closed Ohm  ROFF_res=R_opened Ohm  Roff_gmin=ee.enum.switches.offResistance.no  ROFF=1e12 Ohm  TD=0 s
      settings: SourceProductBaseCode=PS  InternalSimscapePortConfiguration="{\"Bottom\":[],\"Left\":[{\"id\":\"p1\",\"label\":\"1+\",\"type\":\"foundation.electrical.electrical\"},{\"id\":\"p2\",\"label\":\"2+\",\"type\":\"foundation.electrical.electrical\"}],\"Right\":[{\"id\":\"n1\",\"label\":\"1-\",\"type\":\"foundation.electrical.electrical\"},{\"id\":\"n2\",\"label\":\"2-\",\"type\":\"foundation.electrical.electrical\"}],\"Top\":[]}"
  Voltage-Controlled Switch1 : ee_lib/Additional Components/SPICE Passives/Voltage-Controlled Switch  SWITCH_model=ee.enum.switches.switchModelVoltage.resistance  VON=0.7 V  VOFF=0.3 V  VT=0 V  VH=0 V  RON=R_closed Ohm  ROFF_res=R_opened Ohm  Roff_gmin=ee.enum.switches.offResistance.no  ROFF=1e12 Ohm  TD=0 s
      settings: SourceProductBaseCode=PS  InternalSimscapePortConfiguration="{\"Bottom\":[],\"Left\":[{\"id\":\"p1\",\"label\":\"1+\",\"type\":\"foundation.electrical.electrical\"},{\"id\":\"p2\",\"label\":\"2+\",\"type\":\"foundation.electrical.electrical\"}],\"Right\":[{\"id\":\"n1\",\"label\":\"1-\",\"type\":\"foundation.electrical.electrical\"},{\"id\":\"n2\",\"label\":\"2-\",\"type\":\"foundation.electrical.electrical\"}],\"Top\":[]}"
  Voltage-Controlled Switch2 : ee_lib/Additional Components/SPICE Passives/Voltage-Controlled Switch  SWITCH_model=ee.enum.switches.switchModelVoltage.resistance  VON=0.7 V  VOFF=0.3 V  VT=0 V  VH=0 V  RON=R_closed Ohm  ROFF_res=R_opened Ohm  Roff_gmin=ee.enum.switches.offResistance.no  ROFF=1e12 Ohm  TD=0 s
      settings: SourceProductBaseCode=PS  InternalSimscapePortConfiguration="{\"Bottom\":[],\"Left\":[{\"id\":\"p1\",\"label\":\"1+\",\"type\":\"foundation.electrical.electrical\"},{\"id\":\"p2\",\"label\":\"2+\",\"type\":\"foundation.electrical.electrical\"}],\"Right\":[{\"id\":\"n1\",\"label\":\"1-\",\"type\":\"foundation.electrical.electrical\"},{\"id\":\"n2\",\"label\":\"2-\",\"type\":\"foundation.electrical.electrical\"}],\"Top\":[]}"
  V_abc_in : PMIOPort  Side=Left
  V_abc_out : PMIOPort  Port=2  Side=Right
  wires:
  Control/1 -> Simulink-PS Converter3/1
  connections:
  Voltage-Controlled Switch1/LConn1 -- Voltage-Controlled Switch/LConn1 -- Controlled Voltage Source/LConn1 -- Voltage-Controlled Switch2/LConn1
  Voltage-Controlled Switch1/RConn1 -- Voltage-Controlled Switch/RConn1 -- Controlled Voltage Source/RConn2 -- Electrical Reference/LConn1 -- Voltage-Controlled Switch2/RConn1
  Simulink-PS Converter3/RConn1 -- Controlled Voltage Source/RConn1
  Voltage-Controlled Switch/RConn2 -- Phase Splitter/RConn1
  Phase Splitter1/RConn1 -- Voltage-Controlled Switch/LConn2
  V_abc_out/RConn1 -- Phase Splitter1/LConn1
  Voltage-Controlled Switch1/LConn2 -- Phase Splitter1/RConn2
  Voltage-Controlled Switch2/LConn2 -- Phase Splitter1/RConn3
  Voltage-Controlled Switch1/RConn2 -- Phase Splitter/RConn2
  Phase Splitter/LConn1 -- V_abc_in/RConn1
  Voltage-Controlled Switch2/RConn2 -- Phase Splitter/RConn3
